simulink model "chap2_2sim"  (R2016b)
settings: Solver=ode15s  StartTime=0.0  StopTime=RunTime  MaxStep=0.1  RelTol=1e-3  EnableMultiTasking=on
settings Model: Creator=Masoud  LastModifiedBy=Hafez
settings DataIOCC: LimitDataPoints=on  SaveFormat=Array
settings OptimizationCC: LifeSpan=inf
settings DebuggingCC: InheritedTsInSrcMsg=none  SFUnexpectedBacktrackingDiag=warning  SFNoUnconditionalDefaultTransitionDiag=warning  SFExecutionAtInitializationDiag=none
settings HardwareCC: ProdBitPerPointer=32  ProdBitPerSizeT=32  ProdBitPerPtrDiffT=32  ProdLargestAtomicFloat=None  ProdIntDivRoundTo=Undefined  ProdEndianess=Unspecified  ProdWordSize=32  ProdHWDeviceType=32-bit Generic
settings ModelReferenceCC: PropagateSignalLabelsOutOfModel=off
settings GRTTargetCC: TargetLangStandard=C89/C90 (ANSI)  GeneratePreprocessorConditionals=Disable all
settings ConfigComp: CovMetricSettings=dw  CovHtmlReporting=on  CovSaveCumulativeToWorkspaceVar=on  CovSaveSingleToWorkspaceVar=on  CovExternalEMLEnable=off

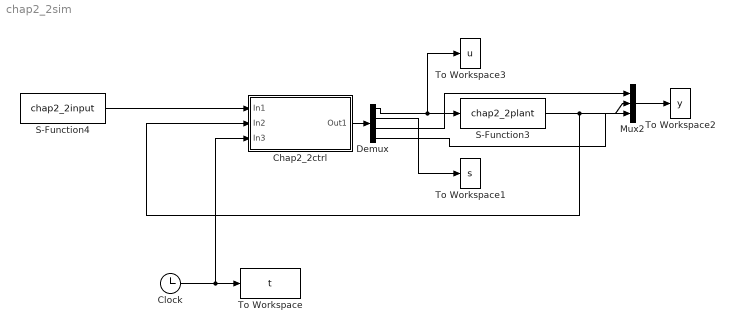
== system chap2_2sim ==
  Chap2_2ctrl : Subsystem
  Clock : Clock
  Demux : Demux
  Mux2 : Mux  Inputs=3
  S-Function3 : S-Function  FunctionName=chap2_2plant  SFunctionModules='chap2_2plant'  SFunctionDeploymentMode=off  EnableBusSupport=off
  S-Function4 : S-Function  FunctionName=chap2_2input  SFunctionModules='chap2_2input'  SFunctionDeploymentMode=off  EnableBusSupport=off
  To Workspace : ToWorkspace  VariableName=t  SampleTime=-1
  To Workspace1 : ToWorkspace  VariableName=s  SampleTime=-1
  To Workspace2 : ToWorkspace  VariableName=y  SampleTime=-1
  To Workspace3 : ToWorkspace  VariableName=u  SampleTime=-1
  wires:
  Clock/1 -> Chap2_2ctrl/3(In3), To Workspace/1
  Mux2/1 -> To Workspace2/1
  Chap2_2ctrl/1(Out1) -> Demux/1
  Demux/1 -> To Workspace3/1, S-Function3/1
  Demux/2 -> To Workspace1/1
  Demux/4 -> Mux2/3
  Demux/3 -> Mux2/1
  S-Function3/1 -> Chap2_2ctrl/2(In2), Mux2/2
  S-Function4/1 -> Chap2_2ctrl/1(In1)

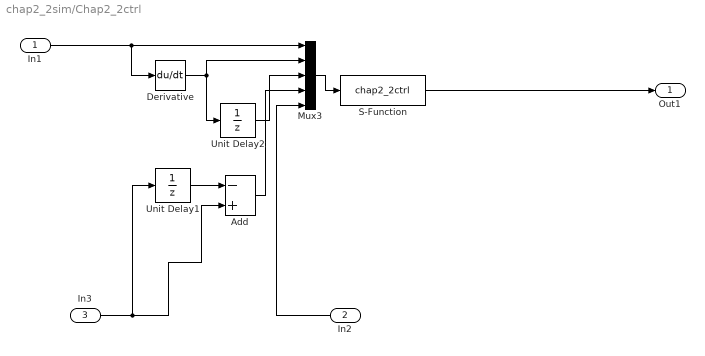
== system chap2_2sim/Chap2_2ctrl ==
  In1 : Inport
  In2 : Inport  Port=2
  In3 : Inport  Port=3
  Add : Sum  Inputs=-+
  Derivative : Derivative
  Mux3 : Mux  Inputs=5
  S-Function : S-Function  FunctionName=chap2_2ctrl  SFunctionModules='chap2_2ctrl'  SFunctionDeploymentMode=off  EnableBusSupport=off
  Unit Delay1 : UnitDelay  SampleTime=-1
  Unit Delay2 : UnitDelay  SampleTime=-1
  Out1 : Outport
  wires:
  S-Function/1 -> Out1/1
  In3/1 -> Add/2, Unit Delay1/1
  In2/1 -> Mux3/5
  Unit Delay2/1 -> Mux3/3
  Derivative/1 -> Mux3/2, Unit Delay2/1
  Mux3/1 -> S-Function/1
  Add/1 -> Mux3/4
  In1/1 -> Derivative/1, Mux3/1
  Unit Delay1/1 -> Add/1
